simulink model "Hopf"  (R2022a)
settings: Solver=FixedStepAuto  StartTime=0.0  StopTime=5  FixedStep=Ts  RelTol=1e-3
values from neighbouring files (symbols this model uses):
  alpha = 10000    [Hopf_oscillator_sim.m]    (also in vdp_forHopf1.m)
  b = 100    [Hopf_oscillator_sim.m]    (also in vdp_forHopf1.m = 1)
  f1 = 0    [Hopf_oscillator_sim.m]    (also in vdp_forHopf1.m)
  f2 = 0    [Hopf_oscillator_sim.m]    (also in vdp_forHopf1.m)
  lamda = 1    [Hopf_oscillator_sim.m]    (also in vdp_forHopf1.m)
  miu = 0.2    [Hopf_oscillator_sim.m]    (also in vdp_forHopf1.m = 1)
  wst = (1-beta)/beta*wsw    (= 5.23598775598)    [Hopf_oscillator_sim.m]    (also in vdp_forHopf1.m)
  wsw = 5*pi    (= 15.7079632679)    [Hopf_oscillator_sim.m]    (also in vdp_forHopf1.m)
undefined symbols (not defined in the file or in its folder): K
settings Model: Creator=suzer  LastModifiedBy=liltrump
settings DebuggingCC: UnconnectedInputMsg=warning  UnconnectedOutputMsg=warning  UnconnectedLineMsg=warning
settings RTWCC: DLArmComputeVersion=19.05

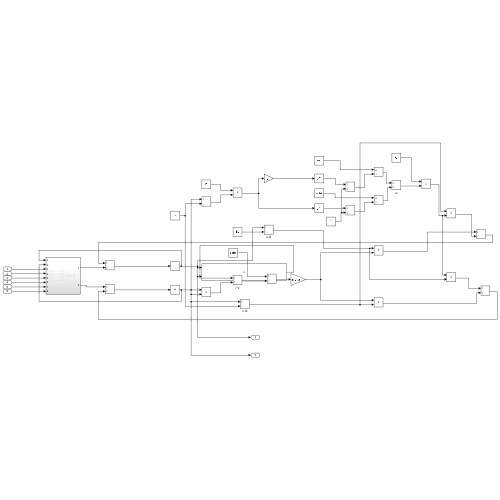
[thumbnail: Simulink's stored preview of the top-level diagram]
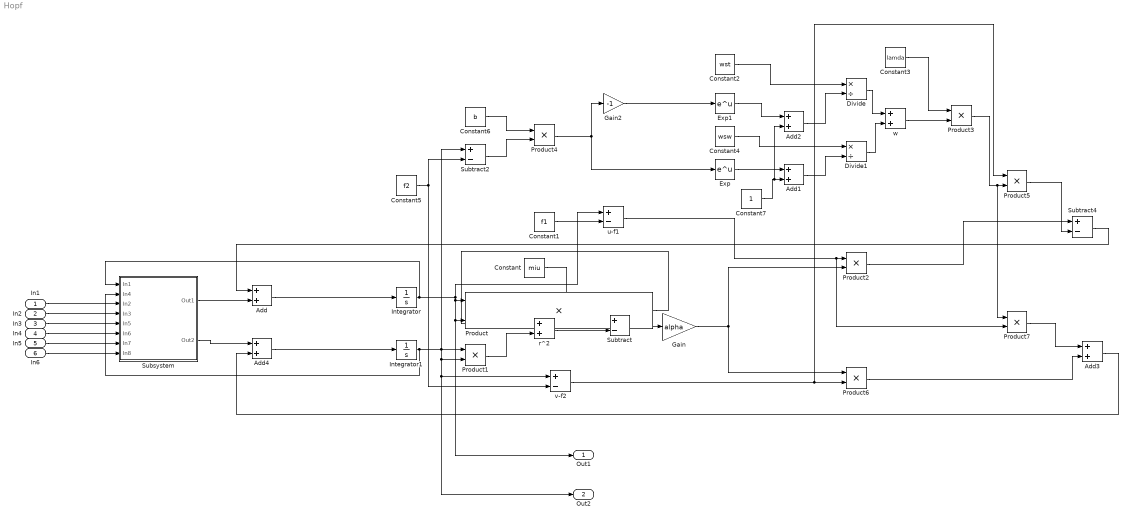
== system Hopf ==
  In1 : Inport
  In2 : Inport  Port=2
  In3 : Inport  Port=3
  In4 : Inport  Port=4
  In5 : Inport  Port=5
  In6 : Inport  Port=6
  Add{,1..4} (5 alike) : Sum
  Constant : Constant  Value=miu
  Constant1 : Constant  Value=f1
  Constant2 : Constant  Value=wst
  Constant3 : Constant  Value=lamda
  Constant4 : Constant  Value=wsw
  Constant5 : Constant  Value=f2
  Constant6 : Constant  Value=b
  Constant7 : Constant
  Divide : Product  Inputs=*/
  Divide1 : Product  Inputs=*/
  Exp : Math
  Exp1 : Math
  Gain : Gain  Gain=alpha
  Gain2 : Gain  Gain=-1
  Integrator : Integrator  InitialCondition=1
  Integrator1 : Integrator
  Product{,1..7} (8 alike) : Product
  Subsystem : Subsystem
  Subtract : Sum  Inputs=+-
  Subtract2 : Sum  Inputs=+-
  Subtract4 : Sum  Inputs=+-
  r^2 : Sum
  u-f1 : Sum  Inputs=+-
  v-f2 : Sum  Inputs=+-
  w : Sum
  Out1 : Outport
  Out2 : Outport  Port=2
  wires:
  Integrator/1 -> Subsystem/1(In1), Product/2, Out1/1, Product/1, u-f1/1
  Integrator1/1 -> Subsystem/2(In4), Out2/1, v-f2/1, Product1/2, Product1/1, Subtract2/1
  Product/1 -> r^2/1
  Product1/1 -> r^2/2
  Constant1/1 -> u-f1/2
  u-f1/1 -> Product7/2, Product2/1
  Constant5/1 -> v-f2/2, Subtract2/2
  Constant6/1 -> Product4/1
  Subtract2/1 -> Product4/2
  Product4/1 -> Exp/1, Gain2/1
  Gain2/1 -> Exp1/1
  Constant2/1 -> Divide/1
  Constant4/1 -> Divide1/1
  Exp/1 -> Add1/1
  Constant7/1 -> Add2/2, Add1/2
  Exp1/1 -> Add2/1
  Add2/1 -> Divide/2
  Add1/1 -> Divide1/2
  Divide/1 -> w/1
  Divide1/1 -> w/2
  w/1 -> Product3/2
  Constant3/1 -> Product3/1
  Constant/1 -> Subtract/1
  r^2/1 -> Subtract/2
  Subtract/1 -> Gain/1
  Gain/1 -> Product6/1, Product2/2
  Product3/1 -> Product7/1, Product5/2
  v-f2/1 -> Product5/1, Product6/2
  Product2/1 -> Subtract4/1
  Product5/1 -> Subtract4/2
  Product7/1 -> Add3/1
  Product6/1 -> Add3/2
  Subtract4/1 -> Add/1
  Add3/1 -> Add4/2
  Subsystem/1(Out1) -> Add/2
  Add/1 -> Integrator/1
  Subsystem/2(Out2) -> Add4/1
  Add4/1 -> Integrator1/1
  In3/1 -> Subsystem/5(In5)
  In4/1 -> Subsystem/6(In6)
  In5/1 -> Subsystem/7(In7)
  In6/1 -> Subsystem/8(In8)
  In1/1 -> Subsystem/3(In2)
  In2/1 -> Subsystem/4(In3)

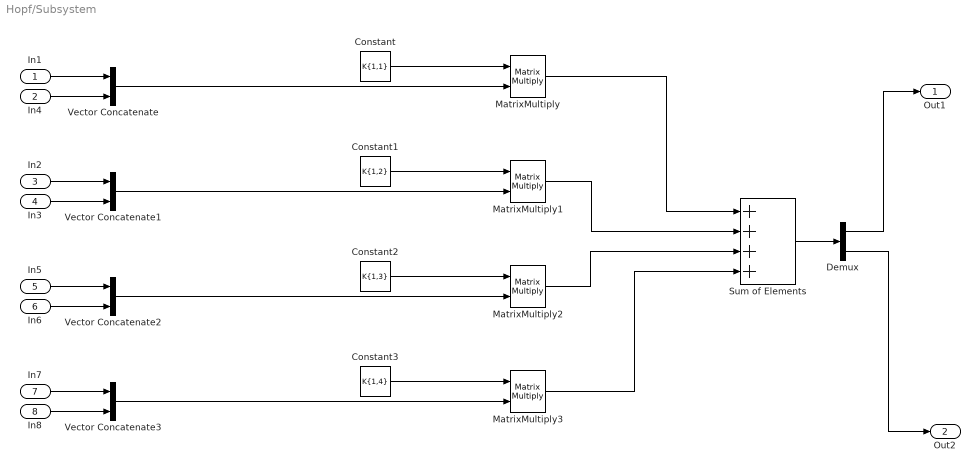
== system Hopf/Subsystem ==
  In1 : Inport
  In4 : Inport  Port=2
  In2 : Inport  Port=3
  In3 : Inport  Port=4
  In5 : Inport  Port=5
  In6 : Inport  Port=6
  In7 : Inport  Port=7
  In8 : Inport  Port=8
  Constant : Constant  Value=K{1,1}  VectorParams1D=off
  Constant1 : Constant  Value=K{1,2}  VectorParams1D=off
  Constant2 : Constant  Value=K{1,3}  VectorParams1D=off
  Constant3 : Constant  Value=K{1,4}  VectorParams1D=off
  Demux : Demux  Outputs=2
  MatrixMultiply{,1..3} (4 alike) : Product  Multiplication=Matrix(*)
  Sum of Elements : Sum  Inputs=++++
  Vector Concatenate{,1..3} (4 alike) : Concatenate
  Out1 : Outport
  Out2 : Outport  Port=2
  wires:
  In1/1 -> Vector Concatenate/1
  Vector Concatenate/1 -> MatrixMultiply/2
  Constant/1 -> MatrixMultiply/1
  Constant1/1 -> MatrixMultiply1/1
  Constant2/1 -> MatrixMultiply2/1
  Constant3/1 -> MatrixMultiply3/1
  MatrixMultiply/1 -> Sum of Elements/1
  MatrixMultiply1/1 -> Sum of Elements/2
  MatrixMultiply2/1 -> Sum of Elements/3
  MatrixMultiply3/1 -> Sum of Elements/4
  Sum of Elements/1 -> Demux/1
  Demux/1 -> Out1/1
  Demux/2 -> Out2/1
  In5/1 -> Vector Concatenate2/1
  In6/1 -> Vector Concatenate2/2
  In7/1 -> Vector Concatenate3/1
  In8/1 -> Vector Concatenate3/2
  Vector Concatenate1/1 -> MatrixMultiply1/2
  Vector Concatenate2/1 -> MatrixMultiply2/2
  Vector Concatenate3/1 -> MatrixMultiply3/2
  In4/1 -> Vector Concatenate/2
  In2/1 -> Vector Concatenate1/1
  In3/1 -> Vector Concatenate1/2
